simulink model "harness_test_system"  (R2024a)
settings: Solver=FixedStepDiscrete  StartTime=0.0  StopTime=0.1  FixedStep=1e-6  RelTol=1e-3
libraries: simulink x2
settings Model: Creator=nmaou  LastModifiedBy=nmaou
settings OptimizationCC: BlockReduction=off  ConditionallyExecuteInputs=off  DefaultParameterBehavior=Inlined
settings DebuggingCC: AlgebraicLoopMsg=error
settings HardwareCC: ProdBitPerPointer=32  ProdBitPerSizeT=32  ProdBitPerPtrDiffT=32  ProdLargestAtomicFloat=None  ProdIntDivRoundTo=Undefined  ProdEndianess=Unspecified  ProdWordSize=32  ProdHWDeviceType=ASIC/FPGA->ASIC/FPGA  TargetBitPerPointer=64  TargetBitPerSizeT=64  TargetBitPerPtrDiffT=64  TargetLongLongMode=on  TargetIntDivRoundTo=Zero  TargetEndianess=LittleEndian  TargetWordSize=64  TargetHWDeviceType=Custom Processor->MATLAB Host Computer  ProdEqTarget=off

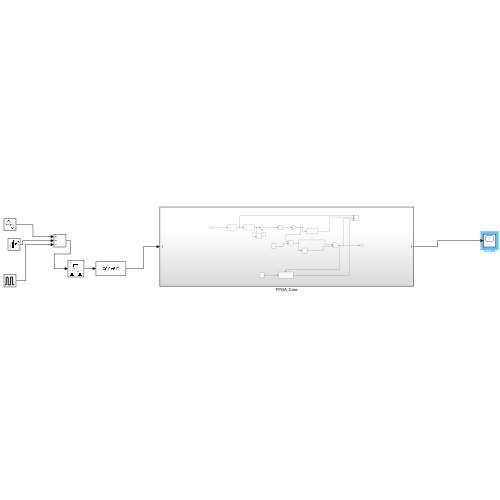
[thumbnail: Simulink's stored preview of the top-level diagram]
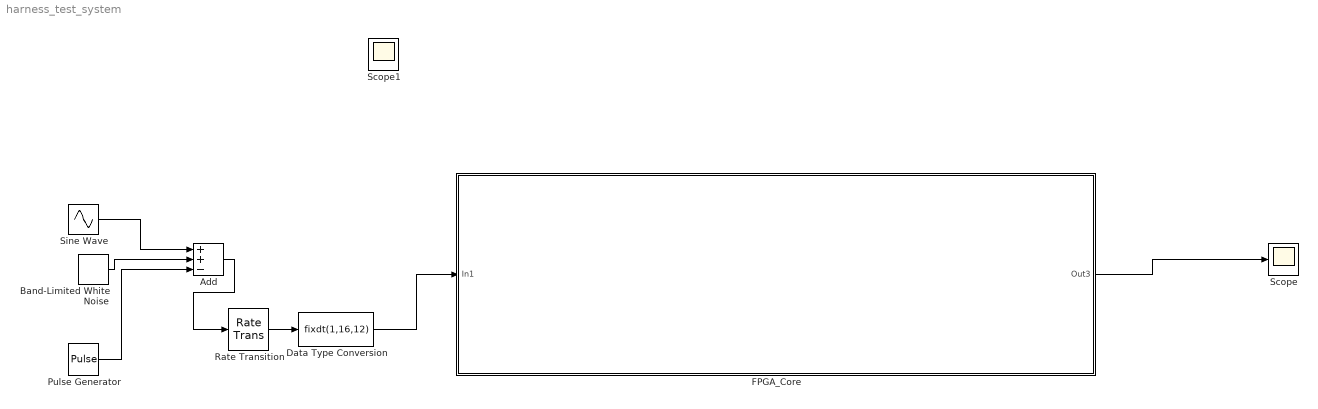
== system harness_test_system ==
  Add : Sum  Inputs=++-
  Band-Limited White Noise : simulink/Sources/Band-Limited White Noise  Cov=[1e-5]  Ts=1e-6  seed=[23341]
  Data Type Conversion : DataTypeConversion  OutDataTypeStr=fixdt(1,16,12)  SaturateOnIntegerOverflow=off  RndMeth=Floor
  FPGA_Core : Subsystem
  Pulse Generator : DiscretePulseGenerator  PulseType=Time based  Amplitude=-2  Period=0.01  PulseWidth=5%  PhaseDelay=0.01
  Rate Transition : RateTransition  OutPortSampleTime=1e-6
  Scope : Scope
  Sine Wave : Sin  Frequency=638.32  SampleTime=1e-6
  Scope1 : Scope
  wires:
  Sine Wave/1 -> Add/1
  Band-Limited White Noise/1 -> Add/2
  Add/1 -> Rate Transition/1
  Data Type Conversion/1 -> FPGA_Core/1(In1)
  Pulse Generator/1 -> Add/3
  Rate Transition/1 -> Data Type Conversion/1
  FPGA_Core/1(Out3) -> Scope/1

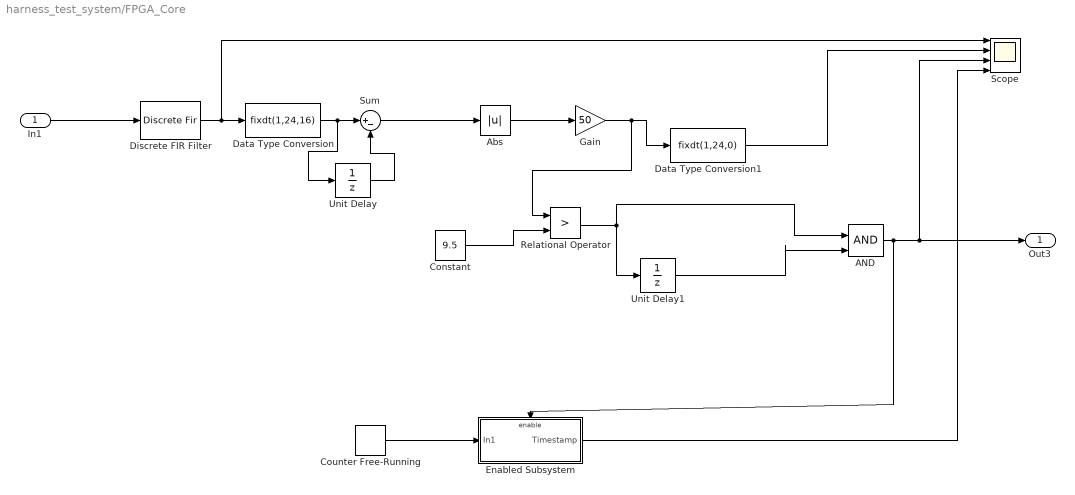
== system harness_test_system/FPGA_Core ==
  In1 : Inport  SampleTime=1e-6
  AND : Logic  IconShape=distinctive  AllPortsSameDT=off  OutDataTypeStr=boolean
  Abs : Abs  SaturateOnIntegerOverflow=off
  Constant : Constant  Value=9.5  OutDataTypeStr=fixdt(1,24,16)  SampleTime=-1
  Counter Free-Running : simulink/Sources/Counter Free-Running  NumBits=32  tsamp=-1
  Data Type Conversion : DataTypeConversion  OutDataTypeStr=fixdt(1,24,16)  RndMeth=Floor
  Data Type Conversion1 : DataTypeConversion  OutDataTypeStr=fixdt(1,24,0)  RndMeth=Floor
  Discrete FIR Filter : DiscreteFir  Coefficients=[0.015625 0.015625 0.015625 0.015625 0.015625 0.015625 0.015625 0.015625 0.015625 0.015625 0.015625 0.015625 0.015625 0.015625 0.015625 0.015625 0.015625 0.015625 0.015625 0.015625 0.015625 0.015625 0.015625 0.015625 0.015625 0.015625 0.015625 0.015625 0.015625 0.015625 0.015625 0.015625 0.015625 0.015625 0.015625 0.015625 0.015625 0.015625 0.015625 0.015625 0.015625 0.015625 0.015625 0.015625 0.015625 0.015625 0.015625 0.015625 0.015625 0.015625 0.015625 0.015625 0.015625 0.015625 0.015625 0.015625 0.015625 0.015625 0.015625 0.015625 0.015625 0.015625 0.015625 0.015625]
  Enabled Subsystem : Subsystem  TreatAsAtomicUnit=on
  Gain : Gain  Gain=50  OutDataTypeStr=fixdt(1,32,20)
  Relational Operator : RelationalOperator  Operator=>  OutDataTypeStr=boolean  RndMeth=Simplest  InputSameDT=off
  Scope : Scope  NumInputPorts=4
  Sum : Sum  Inputs=|+-
  Unit Delay : UnitDelay  SampleTime=-1  HasFrameUpgradeWarning=on
  Unit Delay1 : UnitDelay  SampleTime=-1  HasFrameUpgradeWarning=on
  Out3 : Outport
  wires:
  Gain/1 -> Relational Operator/1, Data Type Conversion1/1
  Unit Delay/1 -> Sum/2
  Sum/1 -> Abs/1
  Abs/1 -> Gain/1
  Relational Operator/1 -> AND/1, Unit Delay1/1
  Counter Free-Running/1 -> Enabled Subsystem/1(In1)
  Data Type Conversion/1 -> Unit Delay/1, Sum/1
  In1/1 -> Discrete FIR Filter/1
  Discrete FIR Filter/1 -> Scope/1, Data Type Conversion/1
  Constant/1 -> Relational Operator/2
  Unit Delay1/1 -> AND/2
  Enabled Subsystem/1(Timestamp) -> Scope/4
  Data Type Conversion1/1 -> Scope/2
  AND/1 -> Scope/3, Out3/1, Enabled Subsystem/Enable

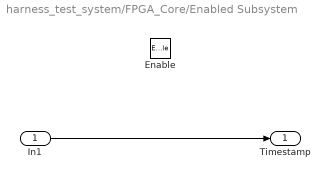
== system harness_test_system/FPGA_Core/Enabled Subsystem ==
  In1 : Inport
  Enable : EnablePort
  Timestamp : Outport
  wires:
  In1/1 -> Timestamp/1
